simulink model "SWC_UDS_type"  (R2021b)
settings: Solver=FixedStepDiscrete  StartTime=0.0  StopTime=10.0  RelTol=1e-3
settings Model: DataDictionary=APPTypes.sldd  Creator=FVT23010  LastModifiedBy=FVT23010
settings DataIOCC: SaveFormat=StructureWithTime
settings OptimizationCC: DefaultParameterBehavior=Inlined  EnhancedBackFolding=on  PassReuseOutputArgsAs=Individual arguments  ZeroExternalMemoryAtStartup=off  ZeroInternalMemoryAtStartup=off  OptimizeBlockOrder=speed  DifferentSizesBufferReuse=on  OptimizationCustomize=off  EfficientTunableParamExpr=on
settings DebuggingCC: ParameterTunabilityLossMsg=error
settings HardwareCC: ProdBitPerPointer=32  ProdBitPerSizeT=32  ProdBitPerPtrDiffT=32  ProdLargestAtomicInteger=Long  ProdLargestAtomicFloat=Double  ProdWordSize=32  ProdLongLongMode=on  ProdHWDeviceType=ARM Compatible->ARM Cortex-M
settings SFSimCC: MATLABDynamicMemAlloc=off
settings RTWCC: Description=AUTOSAR  SystemTargetFile=autosar.tlc  GenCodeOnly=on  TemplateMakefile=ert_default_tmf  PortableWordSizes=on
settings CodeAppCC: ForceParamTrailComments=on  IgnoreCustomStorageClasses=off  OperatorAnnotations=on  SimulinkDataObjDesc=on  SFDataObjDesc=on  InsertBlockDesc=on
settings STFCustomTargetCC: TargetLangStandard=C99 (ISO)  MultiwordLength=256  ParMdlRefBuildCompliant=on  CompOptLevelCompliant=on  IncludeMdlTerminateFcn=off  CombineOutputUpdateFcns=on  SuppressErrorStatus=on  ERTCustomFileBanners=on  SupportNonFinite=off  SupportComplex=off  SupportContinuousTime=off  SupportNonInlinedSFcns=off  RemoveResetFunc=on  MATLABClassNameForMDSCustomization=Simulink.SoftwareTarget.ERTCustomization  AutosarCompliant=on  GRTInterface=off  UseToolchainInfoCompliant=on  LookupTableObjectStructAxisOrder=2,1,3,4,...  LUTObjectStructOrderEvenSpacing=Size,Table,Breakpoints  SystemTargetFile=autosar.tlc
settings ERTTargetCC: TargetLangStandard=C99 (ISO)  ConcurrentExecutionCompliant=off  IncludeMdlTerminateFcn=off  SuppressErrorStatus=on  SupportNonFinite=off  SupportComplex=off  ModelStepFunctionPrototypeControlCompliant=off  CPPClassGenCompliant=off  AutosarCompliant=on  LookupTableObjectStructAxisOrder=2,1,3,4,...  LUTObjectStructOrderEvenSpacing=Size,Table,Breakpoints  GenerateASAP2=on  InlinedParameterPlacement=NonHierarchical  ERTCustomFileTemplate=example_file_process.tlc  ConvertIfToSwitch=off  SuppressUnreachableDefaultCases=off  BooleanTrueId=true_MatlabRTW  BooleanFalseId=false_MatlabRTW

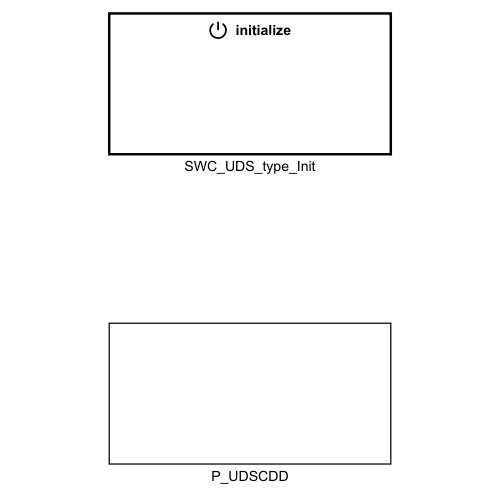
[thumbnail: Simulink's stored preview of the top-level diagram]
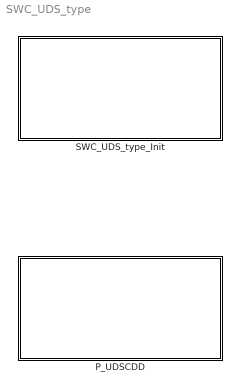
== system SWC_UDS_type ==
  P_UDSCDD : Subsystem
  SWC_UDS_type_Init : Subsystem

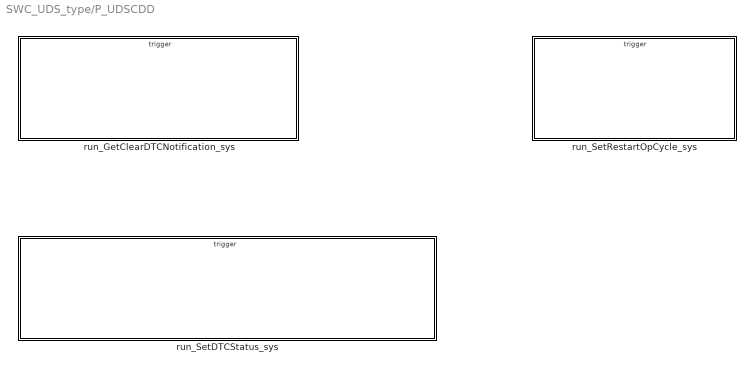
== system SWC_UDS_type/P_UDSCDD ==
  run_GetClearDTCNotification_sys : Subsystem
  run_SetDTCStatus_sys : Subsystem
  run_SetRestartOpCycle_sys : Subsystem

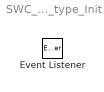
== system SWC_UDS_type/SWC_UDS_type_Init ==
  Event Listener : EventListener  EventName=reset

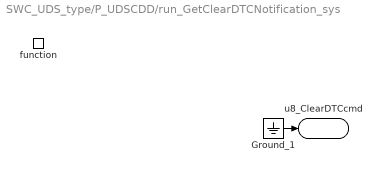
== system SWC_UDS_type/P_UDSCDD/run_GetClearDTCNotification_sys ==
  function : TriggerPort  TriggerType=function-call  IsSimulinkFunction=on  FunctionName=run_GetClearDTCNotification  VariantControl=(inherit)
  Ground_1 : Ground
  u8_ClearDTCcmd : ArgOut  OutDataTypeStr=uint8  ArgumentName=u8_ClearDTCcmd
  wires:
  Ground_1/1 -> u8_ClearDTCcmd/1

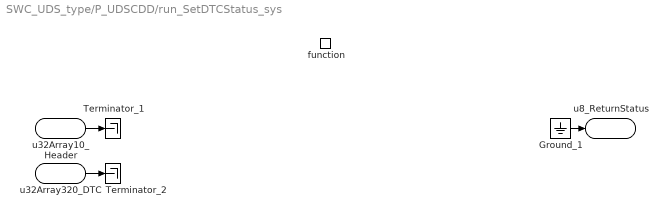
== system SWC_UDS_type/P_UDSCDD/run_SetDTCStatus_sys ==
  function : TriggerPort  TriggerType=function-call  IsSimulinkFunction=on  FunctionName=run_SetDTCStatus  VariantControl=(inherit)
  Ground_1 : Ground
  Terminator_1 : Terminator
  Terminator_2 : Terminator
  u32Array10_Header : ArgIn  OutDataTypeStr=uint32  PortDimensions=10  ArgumentName=u32Array10_Header
  u32Array320_DTC : ArgIn  Port=2  OutDataTypeStr=uint32  PortDimensions=320  ArgumentName=u32Array320_DTC
  u8_ReturnStatus : ArgOut  OutDataTypeStr=uint8  ArgumentName=u8_ReturnStatus
  wires:
  u32Array10_Header/1 -> Terminator_1/1
  u32Array320_DTC/1 -> Terminator_2/1
  Ground_1/1 -> u8_ReturnStatus/1

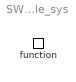
== system SWC_UDS_type/P_UDSCDD/run_SetRestartOpCycle_sys ==
  function : TriggerPort  TriggerType=function-call  IsSimulinkFunction=on  FunctionName=run_SetRestartOpCycle  VariantControl=(inherit)
